simulink model "afe_dq_inv_psm"  (R2025a)
settings: Solver=ode1be  StartTime=0.0  StopTime=simlength  FixedStep=tc  MaxStep=tc
values from neighbouring files (symbols this model uses):
  Adrso = eye(2) + Arso*ts_afe    [init_model.m]
  b = tau_bez/omega_m_bez    [init_model.m]
  Crso = [1 0]    [init_model.m]
  CTRPIFF_CLIP_RELEASE = 0.001    [init_model.m]
  dead_time_AFE = 3e-6    (= 3e-06)    [init_model.m]
  dead_time_INV = 3e-6    (= 3e-06)    [init_model.m]
  deepNEGeta = 0.5    [init_model.m]
  deepNEGxi = 0    [init_model.m]
  deepPOSxi = 0.5    [init_model.m]
  emf_fb_p = 0.2    [init_model.m]
  emf_fb_p_ccaller_1 = emf_fb_p    (= 0.2)    [init_model.m]
  emf_fb_p_ccaller_2 = emf_fb_p    (= 0.2)    [init_model.m]
  emf_p = emf_fb_p*4/10    (= 0.08)    [init_model.m]
  emf_p_ccaller_1 = emf_fb_p_ccaller_1*4/10    (= 0.08)    [init_model.m]
  emf_p_ccaller_2 = emf_fb_p_ccaller_2*4/10    (= 0.08)    [init_model.m]
  fPWM_AFE = 4e3    (= 4000)    [init_model.m]
  fPWM_INV = fPWM_AFE    (= 4000)    [init_model.m]
  g0_500Hz = fcut_500Hz_flt * ts_afe * 2*pi    (= 0.392699081699)    [init_model.m]
  g1_500Hz = 1 - g0_500Hz    (= 0.607300918301)    [init_model.m]
  id_lim = 0.35    [init_model.m]
  Igrid_phase_normalization_factor = 270*sqrt(2)    [grid_emulator.m]    (also in init_model.m = 250e3/Vphase2/3/0.9*sqrt(2))
  iq_lim = 1.4    [init_model.m]
  ixi_pos_ref_lim = 1.6    [init_model.m]
  kg = Kobs(1)    [init_model.m]
  ki_afe = 45    [init_model.m]
  ki_i = 18    [init_model.m]
  ki_rc_grid = 35    [init_model.m]
  ki_vs = 35    [init_model.m]
  ki_w = 18    [init_model.m]
  kp_afe = 0.6    [init_model.m]
  kp_i = 0.25    [init_model.m]
  kp_rc_grid = 0.35    [init_model.m]
  kp_vs = 0.85    [init_model.m]
  kp_w = 2.5    [init_model.m]
  kw = Kobs(2)    [init_model.m]
  Ldrso = acker(Adrso',Crso',polesdrso)'    [init_model.m]
  motorc_m_scale = 2/3*Vdc_bez/ubez    [init_model.m]
  n1 = rms_perios/f_grid/ts_afe    [init_model.m]
  n10 = rms_perios/f_grid/ts_afe    [init_model.m]
  omega_grid_emulator_nom = w_grid    (= 314.159265359)    [grid_emulator.m]
  omega_grid_nom = w_grid    (= 314.159265359)    [grid_emulator.m]
  omega_m_sim = omega_m_bez    [init_model.m]
  pll_i1 = 80    [init_model.m]
  pll_i1_ddsrt = pll_i1/2    (= 40)    [init_model.m]
  pll_p = 1    [init_model.m]
  pll_p_ddsrt = pll_p/2    (= 0.5)    [init_model.m]
  pll_p_frt = 0.2    [init_model.m]
  simlength = 2    [init_model.m]
  start_time_LVRT = 2.0    (= 2)    [init_model.m]
  tc = ts_afe/200    (= 6.25e-07)    [init_model.m]
  time_aux_power_supply_fault = 1e3    (= 1000)    [init_model.m]
  time_phase_fault = 1e3    (= 1000)    [init_model.m]
  time_start_motor_control = 0.035    [init_model.m]
  ts_afe = 1/fPWM_AFE/2    (= 0.000125)    [init_model.m]
  ts_inv = 1/fPWM_INV/2    (= 0.000125)    [init_model.m]
  ugrid_factor = 1    [grid_emulator.m]
  V_phase_normalization_factor = Vgrid_phase_normalization_factor    [grid_emulator.m]
  Vdc_bez = 1070    [grid_emulator.m]
  Vdc_norm_ref = Vdc_ref/Vdc_nom    [init_model.m]
  Vdc_ref = 1070    [init_model.m]
  Vemu_ref_norm = Vemu_ref * sqrt(2) / V_phase_normalization_factor    [grid_emulator.m]
  Vgrid_phase_normalization_factor = Vphase2*sqrt(2)    [grid_emulator.m]    (also in init_model.m)
  vn_eta_pu = 0    [grid_emulator.m]
  vn_xi_pu = 0    [grid_emulator.m]
  vp_xi_pu = 1    [grid_emulator.m]
undefined symbols (not defined in the file or in its folder): Amplitude_U, Amplitude_V, Amplitude_W, end_time_LVRT, ibez, Jm, Ld_norm, Lq_norm, Ls_norm, magnitude, omega_bez, omega_m_bez, Phase_shift, psi_bez, psi_m, psi_m_norm, rpm_bez, rpm_torque_curve, Rs_norm, t_ramp, tau_bez, torque_torque_curve
libraries: fl_lib x114, nesl_utility x78, cstblocks x14, single_phase_transformer_lib x3, threephase_inductor_lib x2, simulink x2, flexshaft_lib x1, pmsm_uvw_with_harmonics_lib x1
(part 1 of 8)
settings Model: SimulationMode=accelerator  Creator=dbagn  LastModifiedBy=dbagn
settings SolverCC: NumberNewtonIterations=3.0  ZeroCrossControl=DisableAll  AlgebraicLoopSolver=TrustRegion  SolverResetMethod=Robust
settings DataIOCC: ReturnWorkspaceOutputs=off
settings OptimizationCC: ReuseModelBlockBuffer=off
settings DebuggingCC: UnconnectedInputMsg=warning  UnconnectedOutputMsg=warning  UnconnectedLineMsg=warning
settings ModelReferenceCC: EnableRefExpFcnMdlSchedulingChecks=on
settings SFSimCC: CustomCodeUndefinedFunction=ThrowError
settings SFSimCC: SimCustomHeaderCode=|
  | #include "mavgflt.h"
  | #include "mavgflt_simulink.h"
  | #include "bemf_obsv.h"
  | #include "bemf_obsv_simulink.h"
  | #include "bemf_obsv_load_est.h"
  | #include "bemf_obsv_load_est_simulink.h"
  | #include "dqvector_pi.h"
  | #include "dqvector_pi_simulink.h"
  | #include "sv_pwm_simulink.h"
  | #include "sv_pwm.h"
  | #include "first_harmonic_tracker.h"
  | #include "first_harmonic_tracker_simulink.h"
  | #include "dqpll_thyr.h"
  | #include "dqpll_thyr_simulink.h"
  | #include "dqpll_grid.h"
  | #include "dqpll_grid_simulink.h"
settings SFSimCC: SimUserSources=|
  | "mavgflt_simulink.c"
  | "mavgflt.c"
  | "bemf_obsv_simulink.c"
  | "bemf_obsv.c"
  | "bemf_obsv_load_est_simulink.c"
  | "bemf_obsv_load_est.c"
  | "dqvector_pi.c"
  | "dqvector_pi_simulink.c"
  | "sv_pwm_simulink.c"
  | "sv_pwm.c"
  | "first_harmonic_tracker_simulink.c"
  | "first_harmonic_tracker.c"
  | "dqpll_thyr_simulink.c"
  | "dqpll_thyr.c"
  | "dqpll_grid_simulink.c"
  | "dqpll_grid.c"
settings SFSimCC: SimUserIncludeDirs=|
  | include
  | src
settings RTWCC: GPUComputeCapability=3.5  DLArmComputeVersion=19.05

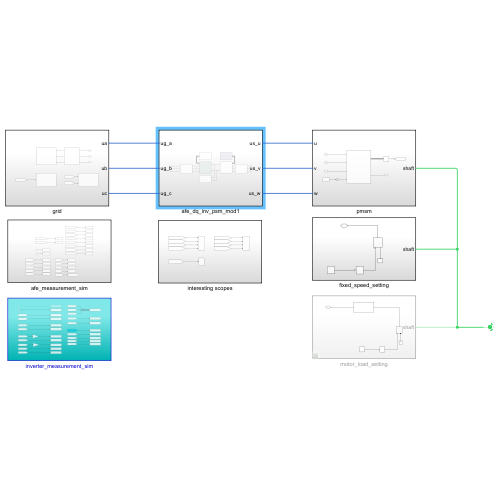
[thumbnail: Simulink's stored preview of the top-level diagram]
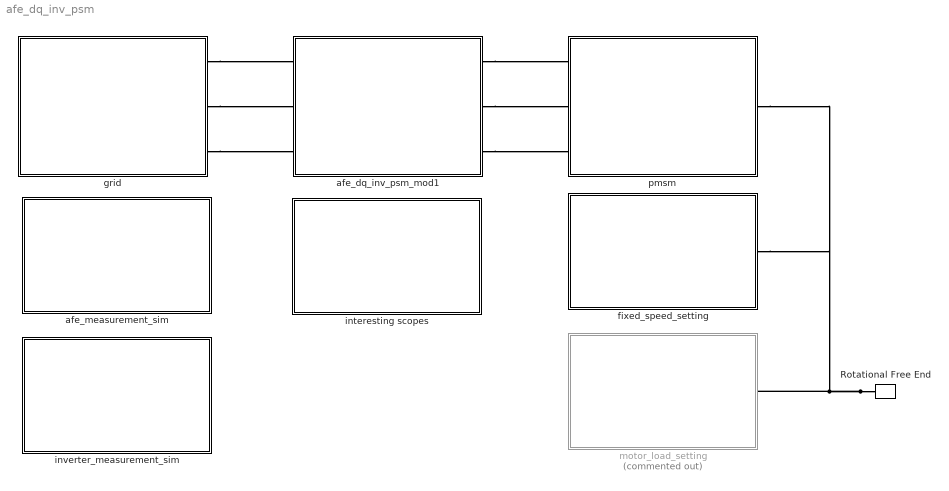
== system afe_dq_inv_psm ==
  Rotational Free End : fl_lib/Mechanical/Rotational Elements/Rotational Free End  w_specify=off  w_priority=None  w=0 rad/s  w_nominal_specify=off  w_nominal_value=1  w_nominal_unit=rad/s
  afe_dq_inv_psm_mod1 : Subsystem
  afe_measurement_sim : Subsystem
  fixed_speed_setting : Subsystem
  grid : Subsystem
  interesting scopes : Subsystem
  inverter_measurement_sim : Subsystem
  motor_load_setting : Subsystem  Commented=on
  pmsm : Subsystem
  connections:
  Rotational Free End/LConn1 -- pmsm/RConn1 -- fixed_speed_setting/LConn1 -- motor_load_setting/LConn1
  grid/RConn1 -- afe_dq_inv_psm_mod1/LConn1
  afe_dq_inv_psm_mod1/RConn1 -- pmsm/LConn1
  grid/RConn2 -- afe_dq_inv_psm_mod1/LConn2
  afe_dq_inv_psm_mod1/RConn2 -- pmsm/LConn2
  grid/RConn3 -- afe_dq_inv_psm_mod1/LConn3
  afe_dq_inv_psm_mod1/RConn3 -- pmsm/LConn3

== system afe_dq_inv_psm/afe_dq_inv_psm_mod1 ==
  LCL_filter : Subsystem
  L_filter : Subsystem
  afe : Subsystem
  afe_control : Subsystem
  brake : Subsystem
  inverter : Subsystem
  inverter_control : Subsystem
  ug_a : PMIOPort  Side=Left
  us_u : PMIOPort  Port=2  Side=Right
  ug_b : PMIOPort  Port=3  Side=Left
  us_v : PMIOPort  Port=4  Side=Right
  ug_c : PMIOPort  Port=5  Side=Left
  us_w : PMIOPort  Port=6  Side=Right
  wires:
  inverter_control/1(uab) -> inverter/1(uab)
  afe_control/1(uab_out) -> afe/1(uab)
  connections:
  L_filter/LConn2 -- inverter/LConn2
  inverter/RConn2 -- brake/LConn2 -- afe/RConn2
  inverter/RConn1 -- brake/LConn1 -- afe/RConn1
  L_filter/LConn1 -- inverter/LConn1
  L_filter/LConn3 -- inverter/LConn3
  L_filter/RConn2 -- us_v/RConn1
  L_filter/RConn3 -- us_w/RConn1
  L_filter/RConn1 -- us_u/RConn1
  LCL_filter/LConn1 -- afe/LConn1
  LCL_filter/LConn2 -- afe/LConn2
  LCL_filter/LConn3 -- afe/LConn3
  ug_a/RConn1 -- LCL_filter/RConn1
  ug_b/RConn1 -- LCL_filter/RConn2
  ug_c/RConn1 -- LCL_filter/RConn3

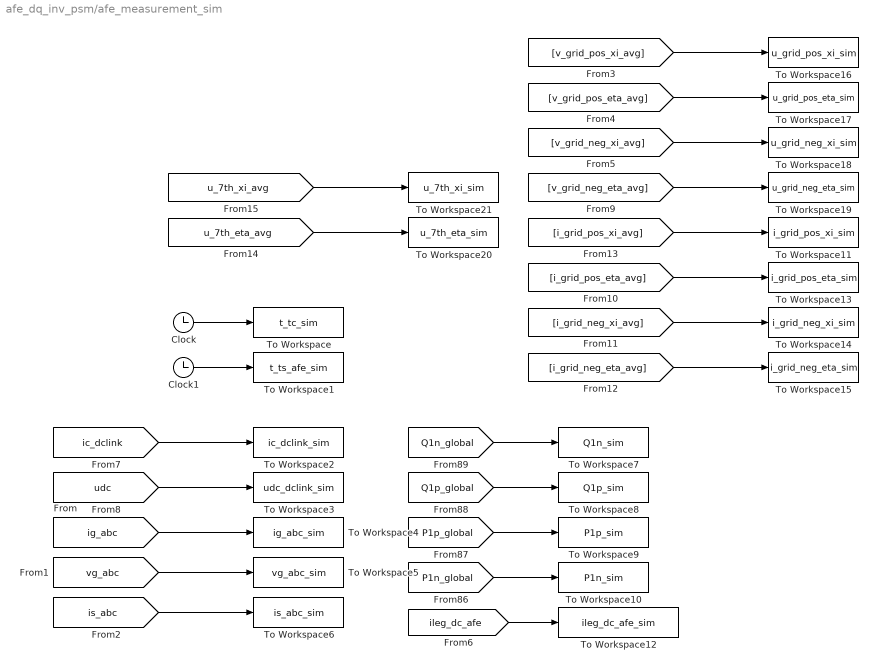
== system afe_dq_inv_psm/afe_measurement_sim ==
  Clock : Clock
  Clock1 : Clock
  To Workspace : ToWorkspace  VariableName=t_tc_sim  SampleTime=tc
      settings: MaxDataPoints=Nc
  To Workspace1 : ToWorkspace  VariableName=t_ts_afe_sim  SampleTime=ts_afe
      settings: MaxDataPoints=Ns_afe
  To Workspace10 : ToWorkspace  VariableName=P1n_sim  SampleTime=ts_afe
      settings: MaxDataPoints=Ns_afe
  To Workspace11 : ToWorkspace  VariableName=i_grid_pos_xi_sim  SampleTime=ts_afe
      settings: MaxDataPoints=Ns_afe
  To Workspace12 : ToWorkspace  VariableName=ileg_dc_afe_sim  SampleTime=tc
      settings: MaxDataPoints=Nc
  To Workspace13 : ToWorkspace  VariableName=i_grid_pos_eta_sim  SampleTime=ts_afe
      settings: MaxDataPoints=Ns_afe
  To Workspace14 : ToWorkspace  VariableName=i_grid_neg_xi_sim  SampleTime=ts_afe
      settings: MaxDataPoints=Ns_afe
  To Workspace15 : ToWorkspace  VariableName=i_grid_neg_eta_sim  SampleTime=ts_afe
      settings: MaxDataPoints=Ns_afe
  To Workspace16 : ToWorkspace  VariableName=u_grid_pos_xi_sim  SampleTime=ts_afe
      settings: MaxDataPoints=Ns_afe
  To Workspace17 : ToWorkspace  VariableName=u_grid_pos_eta_sim  SampleTime=ts_afe
      settings: MaxDataPoints=Ns_afe
  To Workspace18 : ToWorkspace  VariableName=u_grid_neg_xi_sim  SampleTime=ts_afe
      settings: MaxDataPoints=Ns_afe
  To Workspace19 : ToWorkspace  VariableName=u_grid_neg_eta_sim  SampleTime=ts_afe
      settings: MaxDataPoints=Ns_afe
  To Workspace2 : ToWorkspace  VariableName=ic_dclink_sim  SampleTime=tc
      settings: MaxDataPoints=Nc
  To Workspace20 : ToWorkspace  VariableName=u_7th_eta_sim  SampleTime=ts_afe
      settings: MaxDataPoints=Ns_afe
  To Workspace21 : ToWorkspace  VariableName=u_7th_xi_sim  SampleTime=ts_afe
      settings: MaxDataPoints=Ns_afe
  To Workspace3 : ToWorkspace  VariableName=udc_dclink_sim  SampleTime=tc
      settings: MaxDataPoints=Nc
  To Workspace4 : ToWorkspace  VariableName=ig_abc_sim  SampleTime=tc
      settings: MaxDataPoints=Nc
  To Workspace5 : ToWorkspace  VariableName=vg_abc_sim  SampleTime=tc
      settings: MaxDataPoints=Nc
  To Workspace6 : ToWorkspace  VariableName=is_abc_sim  SampleTime=tc
      settings: MaxDataPoints=Nc
  To Workspace7 : ToWorkspace  VariableName=Q1n_sim  SampleTime=ts_afe
      settings: MaxDataPoints=Ns_afe
  To Workspace8 : ToWorkspace  VariableName=Q1p_sim  SampleTime=ts_afe
      settings: MaxDataPoints=Ns_afe
  To Workspace9 : ToWorkspace  VariableName=P1p_sim  SampleTime=ts_afe
      settings: MaxDataPoints=Ns_afe
  wires:
  Clock1/1 -> To Workspace1/1
  Clock/1 -> To Workspace/1
  [ic_dclink] -> To Workspace2/1
  [udc] -> To Workspace3/1
  [ig_abc] -> To Workspace4/1
  [vg_abc] -> To Workspace5/1
  [is_abc] -> To Workspace6/1
  [Q1n_global] -> To Workspace7/1
  [Q1p_global] -> To Workspace8/1
  [P1p_global] -> To Workspace9/1
  [P1n_global] -> To Workspace10/1
  [ileg_dc_afe] -> To Workspace12/1
  [i_grid_pos_xi_avg] -> To Workspace11/1
  [i_grid_pos_eta_avg] -> To Workspace13/1
  [i_grid_neg_xi_avg] -> To Workspace14/1
  [i_grid_neg_eta_avg] -> To Workspace15/1
  [v_grid_pos_xi_avg] -> To Workspace16/1
  [v_grid_pos_eta_avg] -> To Workspace17/1
  [v_grid_neg_xi_avg] -> To Workspace18/1
  [v_grid_neg_eta_avg] -> To Workspace19/1
  [u_7th_eta_avg] -> To Workspace20/1
  [u_7th_xi_avg] -> To Workspace21/1

== system afe_dq_inv_psm/fixed_speed_setting ==
  Ideal Angular Velocity Source : fl_lib/Mechanical/Mechanical Sources/Ideal Angular Velocity Source
  Mechanical Rotational Reference : fl_lib/Mechanical/Rotational Elements/Mechanical Rotational Reference
  PS Step1 : fl_lib/Physical Signals/Sources/PS Step  step_time=0.025 s  initial_value=0 rpm  final_value=rpm_sim rpm
  PS Transfer Function : fl_lib/Physical Signals/Linear Operators/PS Transfer Function  transfer_function_type=foundation.enum.transfer_function_type.lag  T=0.1 s  T1=2 s  T2=1 s  reset_method=foundation.enum.IntegratorResetSpec.None  initial_condition_spec=foundation.enum.IntegratorICSpec.Internal  y0=0 rpm
      settings: InternalSimscapePortConfiguration="{\"Bottom\":[],\"Left\":[{\"id\":\"U\",\"label\":\"\",\"type\":\"input\"}],\"Right\":[{\"id\":\"Y\",\"label\":\"\",\"type\":\"output\"}],\"Top\":[]}"
  shaft : PMIOPort  Side=Left
  connections:
  Mechanical Rotational Reference/LConn1 -- Ideal Angular Velocity Source/RConn2
  Ideal Angular Velocity Source/LConn1 -- shaft/RConn1
  PS Step1/RConn1 -- PS Transfer Function/LConn1
  PS Transfer Function/RConn1 -- Ideal Angular Velocity Source/RConn1

== system afe_dq_inv_psm/grid ==
  grid_emulator : Subsystem
  instantaneus_power : Subsystem
  sequences : Subsystem
  threephase_vi_measures : Subsystem
  ua : PMIOPort  Side=Right
  ub : PMIOPort  Port=2  Side=Right
  uc : PMIOPort  Port=3  Side=Right
  wires:
  [gamma_grid_pll] -> sequences/1(wt)
  [vg_abc] -> instantaneus_power/1(Vline)
  [ig_abc] -> instantaneus_power/2(Iline)
  connections:
  threephase_vi_measures/LConn3 -- grid_emulator/RConn3
  threephase_vi_measures/LConn1 -- grid_emulator/RConn1
  threephase_vi_measures/RConn2 -- ub/RConn1
  threephase_vi_measures/LConn2 -- grid_emulator/RConn2
  threephase_vi_measures/RConn1 -- ua/RConn1
  threephase_vi_measures/RConn3 -- uc/RConn1

== system afe_dq_inv_psm/interesting scopes ==
  current_sequences : Scope  NumInputPorts=4
      settings: SampleTime=ts_afe  ActiveDisplayYMinimum=-1.81849  ActiveDisplayYMaximum=0.36458  DataLoggingVariableName=ScopeData2
  i_grid_seq_ref : Scope
      settings: SampleTime=ts_afe  ActiveDisplayYMinimum=-1.125  ActiveDisplayYMaximum=0.125
  voltage_sequences : Scope  NumInputPorts=4
      settings: SampleTime=ts_afe  ActiveDisplayYMinimum=-0.75427  ActiveDisplayYMaximum=1.21467
  wires:
  [v_grid_neg_eta_avg] -> voltage_sequences/4  "u_grid_neg_eta"
  [i_grid_neg_xi_avg] -> current_sequences/3  "i_grid_neg_xi"
  [v_grid_pos_eta_avg] -> voltage_sequences/2  "u_grid_pos_eta"
  [v_grid_neg_xi_avg] -> voltage_sequences/3  "u_grid_neg_xi"
  [i_grid_pos_xi_avg] -> current_sequences/1  "i_grid_pos_xi"
  [i_grid_neg_eta_avg] -> current_sequences/4  "i_grid_neg_eta"
  [v_grid_pos_xi_avg] -> voltage_sequences/1  "u_grid_pos_xi"
  [i_grid_pos_eta_avg] -> current_sequences/2  "i_grid_pos_eta"
  [i_grid_seq_ref] -> i_grid_seq_ref/1  "i_grid_seq_ref"

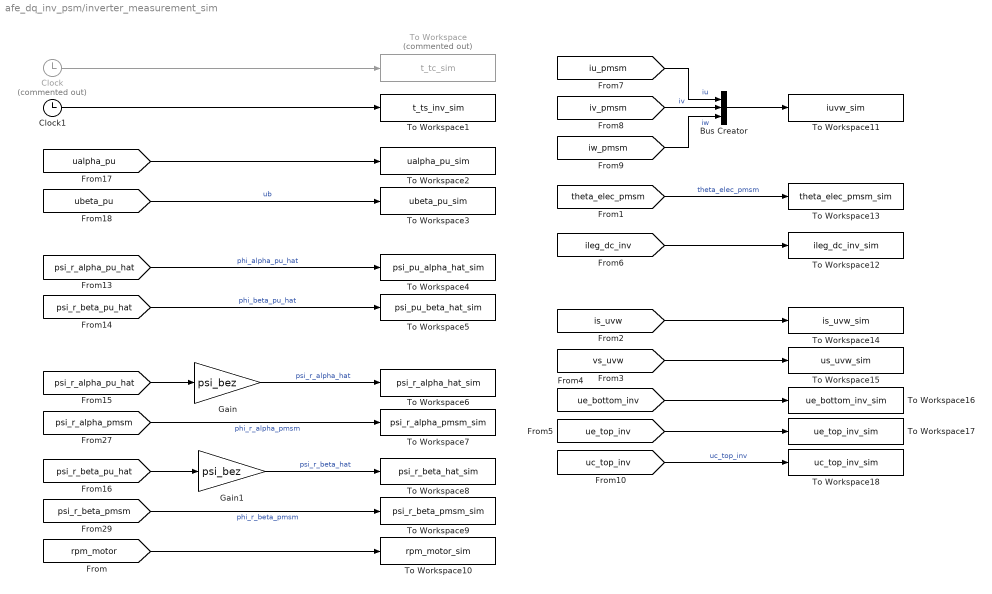
== system afe_dq_inv_psm/inverter_measurement_sim ==
  Bus Creator : BusCreator  Inputs=3
  Clock : Clock  Commented=on
  Clock1 : Clock
  Gain : Gain  Gain=psi_bez
  Gain1 : Gain  Gain=psi_bez
  To Workspace : ToWorkspace  Commented=on  VariableName=t_tc_sim  SampleTime=tc
      settings: MaxDataPoints=Nc
  To Workspace1 : ToWorkspace  VariableName=t_ts_inv_sim  SampleTime=ts_inv
      settings: MaxDataPoints=Ns_inv
  To Workspace10 : ToWorkspace  VariableName=rpm_motor_sim  SampleTime=ts_inv
      settings: MaxDataPoints=Ns_inv
  To Workspace11 : ToWorkspace  VariableName=iuvw_sim  SampleTime=tc
      settings: MaxDataPoints=Nc
  To Workspace12 : ToWorkspace  VariableName=ileg_dc_inv_sim  SampleTime=tc
      settings: MaxDataPoints=Nc
  To Workspace13 : ToWorkspace  VariableName=theta_elec_pmsm_sim  SampleTime=ts_inv
      settings: MaxDataPoints=Ns_inv
  To Workspace14 : ToWorkspace  VariableName=is_uvw_sim  SampleTime=tc
      settings: MaxDataPoints=Nc
  To Workspace15 : ToWorkspace  VariableName=us_uvw_sim  SampleTime=tc
      settings: MaxDataPoints=Nc
  To Workspace16 : ToWorkspace  VariableName=ue_bottom_inv_sim  SampleTime=tc
      settings: MaxDataPoints=Nc
  To Workspace17 : ToWorkspace  VariableName=ue_top_inv_sim  SampleTime=tc
      settings: MaxDataPoints=Nc
  To Workspace18 : ToWorkspace  VariableName=uc_top_inv_sim  SampleTime=tc
      settings: MaxDataPoints=Nc
  To Workspace2 : ToWorkspace  VariableName=ualpha_pu_sim  SampleTime=ts_inv
      settings: MaxDataPoints=Ns_inv
  To Workspace3 : ToWorkspace  VariableName=ubeta_pu_sim  SampleTime=ts_inv
      settings: MaxDataPoints=Ns_inv
  To Workspace4 : ToWorkspace  VariableName=psi_pu_alpha_hat_sim  SampleTime=ts_inv
      settings: MaxDataPoints=Ns_inv
  To Workspace5 : ToWorkspace  VariableName=psi_pu_beta_hat_sim  SampleTime=ts_inv
      settings: MaxDataPoints=Ns_inv
  To Workspace6 : ToWorkspace  VariableName=psi_r_alpha_hat_sim  SampleTime=ts_inv
      settings: MaxDataPoints=Ns_inv
  To Workspace7 : ToWorkspace  VariableName=psi_r_alpha_pmsm_sim  SampleTime=ts_inv
      settings: MaxDataPoints=Ns_inv
  To Workspace8 : ToWorkspace  VariableName=psi_r_beta_hat_sim  SampleTime=ts_inv
      settings: MaxDataPoints=Ns_inv
  To Workspace9 : ToWorkspace  VariableName=psi_r_beta_pmsm_sim  SampleTime=ts_inv
      settings: MaxDataPoints=Ns_inv
  wires:
  [psi_r_beta_pu_hat] -> Gain1/1
  Gain1/1 -> To Workspace8/1  "psi_r_beta_hat"
  [psi_r_beta_pu_hat] -> To Workspace5/1  "phi_beta_pu_hat"
  [psi_r_alpha_pu_hat] -> To Workspace4/1  "phi_alpha_pu_hat"
  [ualpha_pu] -> To Workspace2/1
  [psi_r_alpha_pmsm] -> To Workspace7/1  "phi_r_alpha_pmsm"
  Clock1/1 -> To Workspace1/1
  Gain/1 -> To Workspace6/1  "psi_r_alpha_hat"
  Clock/1 -> To Workspace/1
  [ubeta_pu] -> To Workspace3/1  "ub"
  [psi_r_alpha_pu_hat] -> Gain/1
  [psi_r_beta_pmsm] -> To Workspace9/1  "phi_r_beta_pmsm"
  [rpm_motor] -> To Workspace10/1
  [iv_pmsm] -> Bus Creator/2  "iv"
  [iw_pmsm] -> Bus Creator/3  "iw"
  [iu_pmsm] -> Bus Creator/1  "iu"
  Bus Creator/1 -> To Workspace11/1
  [theta_elec_pmsm] -> To Workspace13/1  "theta_elec_pmsm"
  [ileg_dc_inv] -> To Workspace12/1
  [is_uvw] -> To Workspace14/1
  [vs_uvw] -> To Workspace15/1
  [ue_bottom_inv] -> To Workspace16/1
  [ue_top_inv] -> To Workspace17/1
  [uc_top_inv] -> To Workspace18/1  "uc_top_inv"

== system afe_dq_inv_psm/motor_load_setting ==
  Ideal Torque Source : fl_lib/Mechanical/Mechanical Sources/Ideal Torque Source
  Mechanical Rotational Reference : fl_lib/Mechanical/Rotational Elements/Mechanical Rotational Reference
  PS Step : fl_lib/Physical Signals/Sources/PS Step  step_time=0.25 s  initial_value=1 N*m  final_value=tau_bez N*m
  PS Transfer Function : fl_lib/Physical Signals/Linear Operators/PS Transfer Function  transfer_function_type=foundation.enum.transfer_function_type.lag  T=1 s  T1=2 s  T2=1 s  reset_method=foundation.enum.IntegratorResetSpec.None  initial_condition_spec=foundation.enum.IntegratorICSpec.Internal  y0=0 N*m
      settings: InternalSimscapePortConfiguration="{\"Bottom\":[],\"Left\":[{\"id\":\"U\",\"label\":\"\",\"type\":\"input\"}],\"Right\":[{\"id\":\"Y\",\"label\":\"\",\"type\":\"output\"}],\"Top\":[]}"
  flex-shaft : Subsystem
      mask Display: disp('flexible shaft')
  shaft : PMIOPort  Side=Left
  connections:
  Ideal Torque Source/LConn1 -- flex-shaft/RConn1
  Ideal Torque Source/RConn2 -- Mechanical Rotational Reference/LConn1
  PS Transfer Function/RConn1 -- Ideal Torque Source/RConn1
  PS Step/RConn1 -- PS Transfer Function/LConn1
  flex-shaft/LConn1 -- shaft/RConn1

== system afe_dq_inv_psm/pmsm ==
  Constant : Constant  Value=psi_m
  Selector : Selector  InputPortWidth=19  IndexOptions=Index vector (dialog)  Indices=16  OutputSizes=1
  Simulink-PS Converter3 : nesl_utility/Simulink-PS Converter  PhysicalDomain=network_engine_domain  SubClassName=ps_input  LeftPortType=input  RightPortType=output  PseudoPeriodic=off  Frequencies=[]  NoiseDistribution=none  NoiseParameters=[]  Unit=V*s  AffineConversion=on  FilteringAndDerivatives=provide  SimscapeFilterOrder=1  InputFilterTimeConstant=0.001  UdotUserProvided=0
  synchronous_motor : Subsystem
  u : PMIOPort  Side=Left
  v : PMIOPort  Port=2  Side=Left
  w : PMIOPort  Port=3  Side=Left
  shaft : PMIOPort  Port=4  Side=Right
  tag scope: rpm_motor=global
  wires:
  synchronous_motor/1(motor_data) -> Selector/1
  Selector/1 -> [rpm_motor]
  Constant/1 -> Simulink-PS Converter3/1
  connections:
  synchronous_motor/LConn1 -- u/RConn1
  Simulink-PS Converter3/RConn1 -- synchronous_motor/LConn4
  synchronous_motor/LConn3 -- w/RConn1
  synchronous_motor/LConn2 -- v/RConn1
  shaft/RConn1 -- synchronous_motor/RConn1

== system afe_dq_inv_psm/afe_dq_inv_psm_mod1/LCL_filter ==
  CFu1 : fl_lib/Electrical/Electrical Elements/Capacitor  c=CFu F  r=RCFu Ohm  g=0 1/Ohm  i_specify=off  i_priority=None  i=0 A  i_nominal_specify=off  i_nominal_value=1  i_nominal_unit=A  v_specify=off  v_priority=None  v=0 V  v_nominal_specify=off  v_nominal_value=1  v_nominal_unit=V  vc_specify=off  vc_priority=High  vc=0 V  vc_nominal_specify=off  vc_nominal_value=1  vc_nominal_unit=V
  CFu2 : fl_lib/Electrical/Electrical Elements/Capacitor  c=CFu F  r=RCFu Ohm  g=0 1/Ohm  i_specify=off  i_priority=None  i=0 A  i_nominal_specify=off  i_nominal_value=1  i_nominal_unit=A  v_specify=off  v_priority=None  v=0 V  v_nominal_specify=off  v_nominal_value=1  v_nominal_unit=V  vc_specify=off  vc_priority=High  vc=0 V  vc_nominal_specify=off  vc_nominal_value=1  vc_nominal_unit=V
  CFu3 : fl_lib/Electrical/Electrical Elements/Capacitor  c=CFu F  r=RCFu Ohm  g=0 1/Ohm  i_specify=off  i_priority=None  i=0 A  i_nominal_specify=off  i_nominal_value=1  i_nominal_unit=A  v_specify=off  v_priority=None  v=0 V  v_nominal_specify=off  v_nominal_value=1  v_nominal_unit=V  vc_specify=off  vc_priority=High  vc=0 V  vc_nominal_specify=off  vc_nominal_value=1  vc_nominal_unit=V
  Inductor : fl_lib/Electrical/Electrical Elements/Inductor  l=1e-6 H  r=0 Ohm  g=1e-9 1/Ohm  i_specify=on  i_priority=High  i=0 A  i_nominal_specify=off  i_nominal_value=1  i_nominal_unit=A  v_specify=off  v_priority=None  v=0 V  v_nominal_specify=off  v_nominal_value=1  v_nominal_unit=V  i_L_specify=off  i_L_priority=High  i_L=0 A  i_L_nominal_specify=off  i_L_nominal_value=1  i_L_nominal_unit=A
  Inductor1 : fl_lib/Electrical/Electrical Elements/Inductor  l=1e-6 H  r=0 Ohm  g=1e-9 1/Ohm  i_specify=on  i_priority=High  i=0 A  i_nominal_specify=off  i_nominal_value=1  i_nominal_unit=A  v_specify=off  v_priority=None  v=0 V  v_nominal_specify=off  v_nominal_value=1  v_nominal_unit=V  i_L_specify=off  i_L_priority=High  i_L=0 A  i_L_nominal_specify=off  i_L_nominal_value=1  i_L_nominal_unit=A
  Inductor2 : fl_lib/Electrical/Electrical Elements/Inductor  l=1e-6 H  r=0 Ohm  g=1e-9 1/Ohm  i_specify=on  i_priority=High  i=0 A  i_nominal_specify=off  i_nominal_value=1  i_nominal_unit=A  v_specify=off  v_priority=None  v=0 V  v_nominal_specify=off  v_nominal_value=1  v_nominal_unit=V  i_L_specify=off  i_L_priority=High  i_L=0 A  i_L_nominal_specify=off  i_L_nominal_value=1  i_L_nominal_unit=A
  threephase inductor : threephase_inductor_lib/threephase inductor  Lp=LFu1_AFE H  L0=LFu1_AFE_0 H  Rp=2.4e-3 Ohm  R0=0.8e-3 Ohm  Lls=5e-6 H  uu_1_specify=off  uu_1_priority=None  uu_1=0 V  uu_1_nominal_specify=off  uu_1_nominal_unit=V  uu_1_nominal_value=1  uv_1_specify=off  uv_1_priority=None  uv_1=0 V  uv_1_nominal_specify=off  uv_1_nominal_unit=V  uv_1_nominal_value=1  uw_1_specify=off  uw_1_priority=None  uw_1=0 V  uw_1_nominal_specify=off  uw_1_nominal_unit=V  uw_1_nominal_value=1  uu_2_specify=off  uu_2_priority=None  uu_2=0 V  uu_2_nominal_specify=off  uu_2_nominal_unit=V  uu_2_nominal_value=1  uv_2_specify=off  uv_2_priority=None  uv_2=0 V  uv_2_nominal_specify=off  uv_2_nominal_unit=V  uv_2_nominal_value=1  uw_2_specify=off  uw_2_priority=None  uw_2=0 V  uw_2_nominal_specify=off  uw_2_nominal_unit=V  uw_2_nominal_value=1  iu_specify=off  iu_priority=High  iu=0 A  iu_nominal_specify=off  iu_nominal_unit=A  iu_nominal_value=1  iv_specify=off  iv_priority=High  iv=0 A  iv_nominal_specify=off  iv_nominal_unit=A  iv_nominal_value=1  iw_specify=off  iw_priority=High  iw=0 A  iw_nominal_specify=off  iw_nominal_unit=A  iw_nominal_value=1
      settings: InternalSimscapePortConfiguration="{\"Bottom\":[],\"Left\":[{\"id\":\"up1\",\"label\":\"u1\",\"type\":\"foundation.electrical.electrical\"},{\"id\":\"vp1\",\"label\":\"v1\",\"type\":\"foundation.electrical.electrical\"},{\"id\":\"wp1\",\"label\":\"w1\",\"type\":\"foundation.electrical.electrical\"}],\"Right\":[{\"id\":\"up2\",\"label\":\"u2\",\"type\":\"foundation.electrical.electrical\"},{\"id\":\"vp2\",\"label\":\"v2\",\"type\":\"foundation.electrical.electrical\"},{\"id\":\"wp2\",\"label\":\"w2\",\"type\":\"foundation.electrical.electrical\"}],\"Top\":[]}"
  threephase_vi_measures_stack : Subsystem
  us_a : PMIOPort  Side=Left
  ug_a : PMIOPort  Port=2  Side=Right
  us_b : PMIOPort  Port=3  Side=Left
  ug_b : PMIOPort  Port=4  Side=Right
  us_c : PMIOPort  Port=5  Side=Left
  ug_c : PMIOPort  Port=6  Side=Right
  connections:
  CFu3/RConn1 -- CFu2/RConn1 -- CFu1/RConn1
  CFu1/LConn1 -- Inductor/RConn1 -- ug_a/RConn1
  ug_c/RConn1 -- Inductor2/RConn1 -- CFu3/LConn1
  CFu2/LConn1 -- Inductor1/RConn1 -- ug_b/RConn1
  threephase_vi_measures_stack/LConn1 -- us_a/RConn1
  threephase_vi_measures_stack/LConn2 -- us_b/RConn1
  threephase_vi_measures_stack/LConn3 -- us_c/RConn1
  threephase_vi_measures_stack/RConn1 -- threephase inductor/LConn1
  threephase_vi_measures_stack/RConn2 -- threephase inductor/LConn2
  threephase_vi_measures_stack/RConn3 -- threephase inductor/LConn3
  threephase inductor/RConn1 -- Inductor/LConn1
  Inductor1/LConn1 -- threephase inductor/RConn2
  Inductor2/LConn1 -- threephase inductor/RConn3

== system afe_dq_inv_psm/afe_dq_inv_psm_mod1/L_filter ==
  Inductor : fl_lib/Electrical/Electrical Elements/Inductor  l=1e-6 H  r=0 Ohm  g=1e-9 1/Ohm  i_specify=off  i_priority=None  i=0 A  i_nominal_specify=off  i_nominal_value=1  i_nominal_unit=A  v_specify=off  v_priority=None  v=0 V  v_nominal_specify=off  v_nominal_value=1  v_nominal_unit=V  i_L_specify=off  i_L_priority=High  i_L=0 A  i_L_nominal_specify=off  i_L_nominal_value=1  i_L_nominal_unit=A
  Inductor1 : fl_lib/Electrical/Electrical Elements/Inductor  l=1e-6 H  r=0 Ohm  g=1e-9 1/Ohm  i_specify=off  i_priority=None  i=0 A  i_nominal_specify=off  i_nominal_value=1  i_nominal_unit=A  v_specify=off  v_priority=None  v=0 V  v_nominal_specify=off  v_nominal_value=1  v_nominal_unit=V  i_L_specify=off  i_L_priority=High  i_L=0 A  i_L_nominal_specify=off  i_L_nominal_value=1  i_L_nominal_unit=A
  Inductor2 : fl_lib/Electrical/Electrical Elements/Inductor  l=1e-6 H  r=0 Ohm  g=1e-9 1/Ohm  i_specify=off  i_priority=None  i=0 A  i_nominal_specify=off  i_nominal_value=1  i_nominal_unit=A  v_specify=off  v_priority=None  v=0 V  v_nominal_specify=off  v_nominal_value=1  v_nominal_unit=V  i_L_specify=off  i_L_priority=High  i_L=0 A  i_L_nominal_specify=off  i_L_nominal_value=1  i_L_nominal_unit=A
  threephase inductor : threephase_inductor_lib/threephase inductor  Lp=LFi H  L0=5e-6 H  Rp=2.4e-3 Ohm  R0=0.8e-3 Ohm  Lls=5e-6 H  uu_1_specify=off  uu_1_priority=None  uu_1=0 V  uu_1_nominal_specify=off  uu_1_nominal_unit=V  uu_1_nominal_value=1  uv_1_specify=off  uv_1_priority=None  uv_1=0 V  uv_1_nominal_specify=off  uv_1_nominal_unit=V  uv_1_nominal_value=1  uw_1_specify=off  uw_1_priority=None  uw_1=0 V  uw_1_nominal_specify=off  uw_1_nominal_unit=V  uw_1_nominal_value=1  uu_2_specify=off  uu_2_priority=None  uu_2=0 V  uu_2_nominal_specify=off  uu_2_nominal_unit=V  uu_2_nominal_value=1  uv_2_specify=off  uv_2_priority=None  uv_2=0 V  uv_2_nominal_specify=off  uv_2_nominal_unit=V  uv_2_nominal_value=1  uw_2_specify=off  uw_2_priority=None  uw_2=0 V  uw_2_nominal_specify=off  uw_2_nominal_unit=V  uw_2_nominal_value=1  iu_specify=off  iu_priority=None  iu=0 A  iu_nominal_specify=off  iu_nominal_unit=A  iu_nominal_value=1  iv_specify=off  iv_priority=None  iv=0 A  iv_nominal_specify=off  iv_nominal_unit=A  iv_nominal_value=1  iw_specify=off  iw_priority=None  iw=0 A  iw_nominal_specify=off  iw_nominal_unit=A  iw_nominal_value=1
      settings: InternalSimscapePortConfiguration="{\"Bottom\":[],\"Left\":[{\"id\":\"up1\",\"label\":\"u1\",\"type\":\"foundation.electrical.electrical\"},{\"id\":\"vp1\",\"label\":\"v1\",\"type\":\"foundation.electrical.electrical\"},{\"id\":\"wp1\",\"label\":\"w1\",\"type\":\"foundation.electrical.electrical\"}],\"Right\":[{\"id\":\"up2\",\"label\":\"u2\",\"type\":\"foundation.electrical.electrical\"},{\"id\":\"vp2\",\"label\":\"v2\",\"type\":\"foundation.electrical.electrical\"},{\"id\":\"wp2\",\"label\":\"w2\",\"type\":\"foundation.electrical.electrical\"}],\"Top\":[]}"
  threephase_vi_measures_stack : Subsystem
  us_u : PMIOPort  Side=Left
  uu : PMIOPort  Port=2  Side=Right
  us_v : PMIOPort  Port=3  Side=Left
  uv : PMIOPort  Port=4  Side=Right
  us_w : PMIOPort  Port=5  Side=Left
  uw : PMIOPort  Port=6  Side=Right
  connections:
  threephase_vi_measures_stack/LConn1 -- us_u/RConn1
  threephase_vi_measures_stack/LConn2 -- us_v/RConn1
  threephase_vi_measures_stack/LConn3 -- us_w/RConn1
  threephase inductor/LConn1 -- threephase_vi_measures_stack/RConn1
  threephase inductor/LConn2 -- threephase_vi_measures_stack/RConn2
  threephase inductor/LConn3 -- threephase_vi_measures_stack/RConn3
  threephase inductor/RConn1 -- Inductor/LConn1
  threephase inductor/RConn2 -- Inductor1/LConn1
  threephase inductor/RConn3 -- Inductor2/LConn1
  Inductor/RConn1 -- uu/RConn1
  Inductor1/RConn1 -- uv/RConn1
  Inductor2/RConn1 -- uw/RConn1

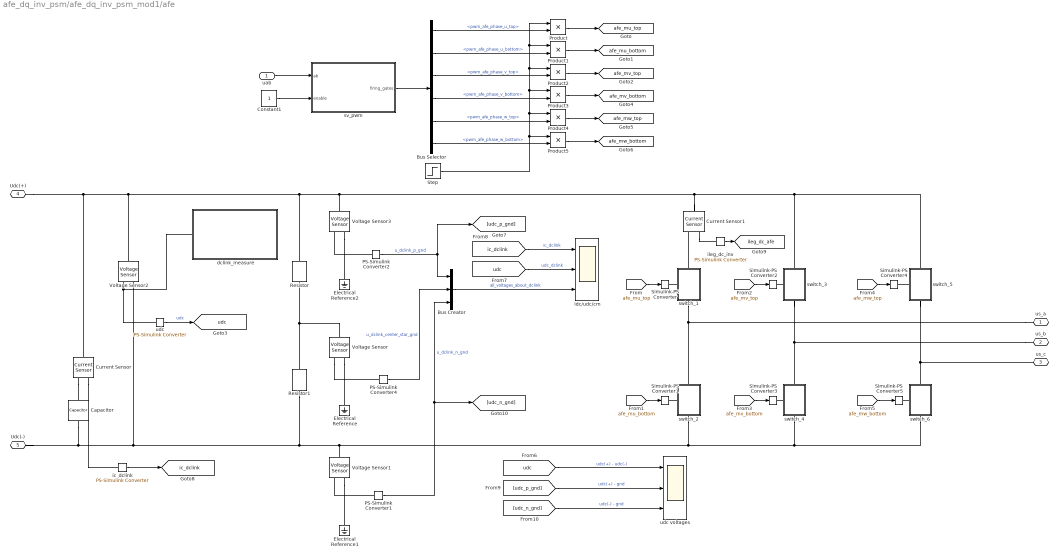
== system afe_dq_inv_psm/afe_dq_inv_psm_mod1/afe ==
  uab : Inport
  Bus Creator : BusCreator  Inputs=3
  Bus Selector : BusSelector  OutputSignals=pwm_afe_phase_u_top,pwm_afe_phase_u_bottom,pwm_afe_phase_v_top,pwm_afe_phase_v_bottom,pwm_afe_phase_w_top,pwm_afe_phase_w_bottom
  Capacitor : fl_lib/Electrical/Electrical Elements/Capacitor  c=CFi F  r=0.2e-3 Ohm  g=0 1/Ohm  i_specify=off  i_priority=None  i=0 A  i_nominal_specify=off  i_nominal_value=1  i_nominal_unit=A  v_specify=on  v_priority=High  v=Vdc_bez V  v_nominal_specify=off  v_nominal_value=1  v_nominal_unit=V  vc_specify=on  vc_priority=High  vc=Vdc_bez V  vc_nominal_specify=off  vc_nominal_value=1  vc_nominal_unit=V
  Constant1 : Constant
  Current Sensor : fl_lib/Electrical/Electrical Sensors/Current Sensor
  Current Sensor1 : fl_lib/Electrical/Electrical Sensors/Current Sensor
  Electrical Reference : fl_lib/Electrical/Electrical Elements/Electrical Reference
  Electrical Reference1 : fl_lib/Electrical/Electrical Elements/Electrical Reference
  Electrical Reference2 : fl_lib/Electrical/Electrical Elements/Electrical Reference
  PS-Simulink Converter1 : nesl_utility/PS-Simulink Converter  PhysicalDomain=network_engine_domain  SubClassName=ps_output  LeftPortType=input  RightPortType=output  PseudoPeriodic=off  Frequencies=[]  VectorFormat=1-D array  Unit=V  AffineConversion=on
  PS-Simulink Converter2 : nesl_utility/PS-Simulink Converter  PhysicalDomain=network_engine_domain  SubClassName=ps_output  LeftPortType=input  RightPortType=output  PseudoPeriodic=off  Frequencies=[]  VectorFormat=1-D array  Unit=V  AffineConversion=on
  PS-Simulink Converter4 : nesl_utility/PS-Simulink Converter  PhysicalDomain=network_engine_domain  SubClassName=ps_output  LeftPortType=input  RightPortType=output  PseudoPeriodic=off  Frequencies=[]  VectorFormat=1-D array  Unit=V  AffineConversion=on
  Product{,1..5} (6 alike) : Product
  Resistor : fl_lib/Electrical/Electrical Elements/Resistor  R=1e6 Ohm  i_specify=off  i_priority=None  i=0 A  i_nominal_specify=off  i_nominal_value=1  i_nominal_unit=A  v_specify=off  v_priority=None  v=0 V  v_nominal_specify=off  v_nominal_value=1  v_nominal_unit=V
  Resistor1 : fl_lib/Electrical/Electrical Elements/Resistor  R=1e6 Ohm  i_specify=off  i_priority=None  i=0 A  i_nominal_specify=off  i_nominal_value=1  i_nominal_unit=A  v_specify=off  v_priority=None  v=0 V  v_nominal_specify=off  v_nominal_value=1  v_nominal_unit=V
  Simulink-PS Converter{,1..5} (6 alike) : nesl_utility/Simulink-PS Converter  PhysicalDomain=network_engine_domain  SubClassName=ps_input  LeftPortType=input  RightPortType=output  PseudoPeriodic=off  Frequencies=[]  NoiseDistribution=none  NoiseParameters=[]  Unit=1  AffineConversion=off  FilteringAndDerivatives=provide  SimscapeFilterOrder=1  InputFilterTimeConstant=0.001  UdotUserProvided=0
  Step : Step  Time=time_aux_power_supply_fault  Before=1  After=0  SampleTime=0
  Voltage Sensor{,1..3} (4 alike) : fl_lib/Electrical/Electrical Sensors/Voltage Sensor
  dclink_measure : Subsystem
  ic_dclink : nesl_utility/PS-Simulink Converter  PhysicalDomain=network_engine_domain  SubClassName=ps_output  LeftPortType=input  RightPortType=output  PseudoPeriodic=off  Frequencies=[]  VectorFormat=1-D array  Unit=A  AffineConversion=on
  idc/udc/cm : Scope  NumInputPorts=3
      settings: SampleTime=tc  ActiveDisplayYMinimum=-1357.19064  ActiveDisplayYMaximum=1822.38118
  ileg_dc_inv : nesl_utility/PS-Simulink Converter  PhysicalDomain=network_engine_domain  SubClassName=ps_output  LeftPortType=input  RightPortType=output  PseudoPeriodic=off  Frequencies=[]  VectorFormat=1-D array  Unit=A  AffineConversion=on
  sv_pwm : Subsystem
  switch_1 : Subsystem
      settings: PortSchema="{\"entries\":[{\"content\":{\"sides\":[{\"content\":{\"connectorIds\":[\"LConn1\"]},\"type\":\"ConnectorPlacement.EquallySpacedRectSide\",\"uuid\":\"9277da8d-d460-43e6-8478-dd662f15d226\"},{\"content\":{\"connectorIds\":[],\"side\":\"RIGHT\"},\"type\":\"ConnectorPlacement.EquallySpacedRectSide\",\"uuid\":\"a7ece396-f1d9-4f4f-a05b-db1fc65d6e1d\"},{\"content\":{\"connectorIds\":[\"LConn2\"],\"side\":\"TOP\"},\"type\":\"ConnectorPlacement.EquallySpacedRectSide\",\"uuid\":\"fdd70777-e9cf-4317-afb6-cae87f75d5b0\"},{\"content\":{\"connectorIds\":[\"RConn1\"],\"side\":\"BOTTOM\"},\"type\":\"ConnectorPlacement.EquallySpacedRectSide\",\"uuid\":\"2353ed68-b1a1-4775-9ca9-31e268d5443b\"}]},\"type\":\"ConnectorPlacement.EquallySpacedConnector\",\"uuid\":\"d5479f4c-4e65-4791-adcb-73df11f88590\"}],\"packageUris\":[\"http://schema.mathworks.com/mf0/Connector/R2020b\"],\"version\":\"1.0\"}"
  switch_2 : Subsystem
      settings: PortSchema="{\"entries\":[{\"content\":{\"sides\":[{\"content\":{\"connectorIds\":[\"LConn1\"]},\"type\":\"ConnectorPlacement.EquallySpacedRectSide\",\"uuid\":\"9277da8d-d460-43e6-8478-dd662f15d226\"},{\"content\":{\"connectorIds\":[],\"side\":\"RIGHT\"},\"type\":\"ConnectorPlacement.EquallySpacedRectSide\",\"uuid\":\"a7ece396-f1d9-4f4f-a05b-db1fc65d6e1d\"},{\"content\":{\"connectorIds\":[\"LConn2\"],\"side\":\"TOP\"},\"type\":\"ConnectorPlacement.EquallySpacedRectSide\",\"uuid\":\"fdd70777-e9cf-4317-afb6-cae87f75d5b0\"},{\"content\":{\"connectorIds\":[\"RConn1\"],\"side\":\"BOTTOM\"},\"type\":\"ConnectorPlacement.EquallySpacedRectSide\",\"uuid\":\"2353ed68-b1a1-4775-9ca9-31e268d5443b\"}]},\"type\":\"ConnectorPlacement.EquallySpacedConnector\",\"uuid\":\"d5479f4c-4e65-4791-adcb-73df11f88590\"}],\"packageUris\":[\"http://schema.mathworks.com/mf0/Connector/R2020b\"],\"version\":\"1.0\"}"
  switch_3 : Subsystem
      settings: PortSchema="{\"entries\":[{\"content\":{\"sides\":[{\"content\":{\"connectorIds\":[\"LConn1\"]},\"type\":\"ConnectorPlacement.EquallySpacedRectSide\",\"uuid\":\"9277da8d-d460-43e6-8478-dd662f15d226\"},{\"content\":{\"connectorIds\":[],\"side\":\"RIGHT\"},\"type\":\"ConnectorPlacement.EquallySpacedRectSide\",\"uuid\":\"a7ece396-f1d9-4f4f-a05b-db1fc65d6e1d\"},{\"content\":{\"connectorIds\":[\"LConn2\"],\"side\":\"TOP\"},\"type\":\"ConnectorPlacement.EquallySpacedRectSide\",\"uuid\":\"fdd70777-e9cf-4317-afb6-cae87f75d5b0\"},{\"content\":{\"connectorIds\":[\"RConn1\"],\"side\":\"BOTTOM\"},\"type\":\"ConnectorPlacement.EquallySpacedRectSide\",\"uuid\":\"2353ed68-b1a1-4775-9ca9-31e268d5443b\"}]},\"type\":\"ConnectorPlacement.EquallySpacedConnector\",\"uuid\":\"d5479f4c-4e65-4791-adcb-73df11f88590\"}],\"packageUris\":[\"http://schema.mathworks.com/mf0/Connector/R2020b\"],\"version\":\"1.0\"}"
  switch_4 : Subsystem
      settings: PortSchema="{\"entries\":[{\"content\":{\"sides\":[{\"content\":{\"connectorIds\":[\"LConn1\"]},\"type\":\"ConnectorPlacement.EquallySpacedRectSide\",\"uuid\":\"9277da8d-d460-43e6-8478-dd662f15d226\"},{\"content\":{\"connectorIds\":[],\"side\":\"RIGHT\"},\"type\":\"ConnectorPlacement.EquallySpacedRectSide\",\"uuid\":\"a7ece396-f1d9-4f4f-a05b-db1fc65d6e1d\"},{\"content\":{\"connectorIds\":[\"LConn2\"],\"side\":\"TOP\"},\"type\":\"ConnectorPlacement.EquallySpacedRectSide\",\"uuid\":\"fdd70777-e9cf-4317-afb6-cae87f75d5b0\"},{\"content\":{\"connectorIds\":[\"RConn1\"],\"side\":\"BOTTOM\"},\"type\":\"ConnectorPlacement.EquallySpacedRectSide\",\"uuid\":\"2353ed68-b1a1-4775-9ca9-31e268d5443b\"}]},\"type\":\"ConnectorPlacement.EquallySpacedConnector\",\"uuid\":\"d5479f4c-4e65-4791-adcb-73df11f88590\"}],\"packageUris\":[\"http://schema.mathworks.com/mf0/Connector/R2020b\"],\"version\":\"1.0\"}"
  switch_5 : Subsystem
      settings: PortSchema="{\"entries\":[{\"content\":{\"sides\":[{\"content\":{\"connectorIds\":[\"LConn1\"]},\"type\":\"ConnectorPlacement.EquallySpacedRectSide\",\"uuid\":\"9277da8d-d460-43e6-8478-dd662f15d226\"},{\"content\":{\"connectorIds\":[],\"side\":\"RIGHT\"},\"type\":\"ConnectorPlacement.EquallySpacedRectSide\",\"uuid\":\"a7ece396-f1d9-4f4f-a05b-db1fc65d6e1d\"},{\"content\":{\"connectorIds\":[\"LConn2\"],\"side\":\"TOP\"},\"type\":\"ConnectorPlacement.EquallySpacedRectSide\",\"uuid\":\"fdd70777-e9cf-4317-afb6-cae87f75d5b0\"},{\"content\":{\"connectorIds\":[\"RConn1\"],\"side\":\"BOTTOM\"},\"type\":\"ConnectorPlacement.EquallySpacedRectSide\",\"uuid\":\"2353ed68-b1a1-4775-9ca9-31e268d5443b\"}]},\"type\":\"ConnectorPlacement.EquallySpacedConnector\",\"uuid\":\"d5479f4c-4e65-4791-adcb-73df11f88590\"}],\"packageUris\":[\"http://schema.mathworks.com/mf0/Connector/R2020b\"],\"version\":\"1.0\"}"
  switch_6 : Subsystem
      settings: PortSchema="{\"entries\":[{\"content\":{\"sides\":[{\"content\":{\"connectorIds\":[\"LConn1\"]},\"type\":\"ConnectorPlacement.EquallySpacedRectSide\",\"uuid\":\"9277da8d-d460-43e6-8478-dd662f15d226\"},{\"content\":{\"connectorIds\":[],\"side\":\"RIGHT\"},\"type\":\"ConnectorPlacement.EquallySpacedRectSide\",\"uuid\":\"a7ece396-f1d9-4f4f-a05b-db1fc65d6e1d\"},{\"content\":{\"connectorIds\":[\"LConn2\"],\"side\":\"TOP\"},\"type\":\"ConnectorPlacement.EquallySpacedRectSide\",\"uuid\":\"fdd70777-e9cf-4317-afb6-cae87f75d5b0\"},{\"content\":{\"connectorIds\":[\"RConn1\"],\"side\":\"BOTTOM\"},\"type\":\"ConnectorPlacement.EquallySpacedRectSide\",\"uuid\":\"2353ed68-b1a1-4775-9ca9-31e268d5443b\"}]},\"type\":\"ConnectorPlacement.EquallySpacedConnector\",\"uuid\":\"d5479f4c-4e65-4791-adcb-73df11f88590\"}],\"packageUris\":[\"http://schema.mathworks.com/mf0/Connector/R2020b\"],\"version\":\"1.0\"}"
  udc : nesl_utility/PS-Simulink Converter  PhysicalDomain=network_engine_domain  SubClassName=ps_output  LeftPortType=input  RightPortType=output  PseudoPeriodic=off  Frequencies=[]  VectorFormat=1-D array  Unit=V  AffineConversion=on
  udc voltages : Scope  NumInputPorts=3
      settings: SampleTime=tc  ActiveDisplayYMinimum=71.02114  ActiveDisplayYMaximum=1379.58028
  us_a : PMIOPort  Side=Left
  us_b : PMIOPort  Port=2  Side=Left
  us_c : PMIOPort  Port=3  Side=Left
  Udc(+) : PMIOPort  Port=4  Side=Right
  Udc(-) : PMIOPort  Port=5  Side=Right
  tag scope: afe_mu_bottom=global, afe_mu_top=global, afe_mv_bottom=global, afe_mv_top=global, afe_mw_bottom=global, afe_mw_top=global, ic_dclink=global, ileg_dc_afe=global, udc=global
  wires:
  uab/1 -> sv_pwm/1(ab)
  [afe_mu_top] -> Simulink-PS Converter/1
  [afe_mu_bottom] -> Simulink-PS Converter1/1
  [afe_mv_top] -> Simulink-PS Converter2/1
  [afe_mv_bottom] -> Simulink-PS Converter3/1
  [afe_mw_top] -> Simulink-PS Converter4/1
  [afe_mw_bottom] -> Simulink-PS Converter5/1
  sv_pwm/1(firing_gates) -> Bus Selector/1
  Constant1/1 -> sv_pwm/2(enable)
  udc/1 -> [udc]  "udc"
  ic_dclink/1 -> [ic_dclink]
  ileg_dc_inv/1 -> [ileg_dc_afe]
  Step/1 -> Product5/1, Product4/1, Product3/1, Product2/1, Product/1, Product1/1
  Bus Selector/1 -> Product/2  "<pwm_afe_phase_u_top>"
  Bus Selector/2 -> Product1/2  "<pwm_afe_phase_u_bottom>"
  Bus Selector/3 -> Product2/2  "<pwm_afe_phase_v_top>"
  Bus Selector/4 -> Product3/2  "<pwm_afe_phase_v_bottom>"
  Bus Selector/5 -> Product4/2  "<pwm_afe_phase_w_top>"
  Bus Selector/6 -> Product5/2  "<pwm_afe_phase_w_bottom>"
  Product/1 -> [afe_mu_top]
  Product1/1 -> [afe_mu_bottom]
  Product2/1 -> [afe_mv_top]
  Product3/1 -> [afe_mv_bottom]
  Product4/1 -> [afe_mw_top]
  Product5/1 -> [afe_mw_bottom]
  [ic_dclink] -> idc/udc/cm/1  "ic_dclink"
  [udc] -> idc/udc/cm/2  "udc_dclink"
  Bus Creator/1 -> idc/udc/cm/3  "all_voltages_about_dclink"
  PS-Simulink Converter2/1 -> [udc_p_gnd], Bus Creator/1  "u_dclink_p_gnd"
  PS-Simulink Converter4/1 -> Bus Creator/2  "u_dclink_center_star_gnd"
  PS-Simulink Converter1/1 -> [udc_n_gnd], Bus Creator/3  "u_dclink_n_gnd"
  [udc_p_gnd] -> udc voltages/2  "udc(+) - gnd"
  [udc_n_gnd] -> udc voltages/3  "udc(-) - gnd"
  [udc] -> udc voltages/1  "udc(+) - udc(-)"
  connections:
  Current Sensor/LConn1 -- Udc(+)/RConn1 -- Voltage Sensor2/LConn1 -- Resistor/LConn1 -- Voltage Sensor3/LConn1 -- Current Sensor1/LConn1 -- switch_5/LConn2 -- switch_3/LConn2
  Udc(-)/RConn1 -- Capacitor/RConn1 -- Voltage Sensor2/RConn2 -- Resistor1/RConn1 -- Voltage Sensor1/LConn1 -- switch_2/RConn1 -- switch_6/RConn1 -- switch_4/RConn1
  switch_1/LConn1 -- Simulink-PS Converter/RConn1
  switch_2/LConn1 -- Simulink-PS Converter1/RConn1
  switch_3/LConn1 -- Simulink-PS Converter2/RConn1
  switch_4/LConn1 -- Simulink-PS Converter3/RConn1
  switch_5/LConn1 -- Simulink-PS Converter4/RConn1
  switch_6/LConn1 -- Simulink-PS Converter5/RConn1
  us_a/RConn1 -- switch_2/LConn2 -- switch_1/RConn1
  us_b/RConn1 -- switch_4/LConn2 -- switch_3/RConn1
  us_c/RConn1 -- switch_6/LConn2 -- switch_5/RConn1
  Voltage Sensor2/RConn1 -- udc/LConn1 -- dclink_measure/LConn1
  Current Sensor/RConn2 -- Capacitor/LConn1
  Current Sensor/RConn1 -- ic_dclink/LConn1
  switch_1/LConn2 -- Current Sensor1/RConn2
  Current Sensor1/RConn1 -- ileg_dc_inv/LConn1
  Resistor1/LConn1 -- Voltage Sensor/LConn1 -- Resistor/RConn1
  Voltage Sensor/RConn2 -- Electrical Reference/LConn1
  Voltage Sensor/RConn1 -- PS-Simulink Converter4/LConn1
  PS-Simulink Converter1/LConn1 -- Voltage Sensor1/RConn1
  Voltage Sensor1/RConn2 -- Electrical Reference1/LConn1
  PS-Simulink Converter2/LConn1 -- Voltage Sensor3/RConn1
  Voltage Sensor3/RConn2 -- Electrical Reference2/LConn1

== system afe_dq_inv_psm/afe_dq_inv_psm_mod1/afe_control ==
  Constant : Constant  Value=Vdc_norm_ref
  current_ctrl : Subsystem
  grid_current_sampling_and_alpha_beta_transformation : Subsystem
  grid_voltage_phase_lock_loops : Subsystem
  grid_voltage_sampling_and_alpha_beta_transformation : Subsystem
  i_alphabeta2xieta : Subsystem
  islanding_mode_detector : Subsystem
  udc_ctrl : Subsystem
  uab_out : Outport
  tag scope: ig_eta_pu=global, ig_xi_pu=global
  wires:
  Constant/1 -> udc_ctrl/2(udc_pu_ref)
  [vdc_pu] -> udc_ctrl/1(udc_pu)
  current_ctrl/1(uab_afe_out) -> uab_out/1
  udc_ctrl/1(i_xi_ref) -> current_ctrl/1(is_xi_ref)  "i_xi_ref"
  [gamma_grid_pll] -> islanding_mode_detector/1(gamma)
  [gamma_grid_pll] -> i_alphabeta2xieta/3(gamma)
  [vg_abc] -> grid_voltage_sampling_and_alpha_beta_transformation/1(v_abc)
  grid_voltage_sampling_and_alpha_beta_transformation/1(u_grid_alpha) -> islanding_mode_detector/2(alpha)
  grid_voltage_sampling_and_alpha_beta_transformation/2(u_grid_beta) -> islanding_mode_detector/3(beta)
  [ig_abc] -> grid_current_sampling_and_alpha_beta_transformation/1(i_abc)
  grid_current_sampling_and_alpha_beta_transformation/1(i_grid_alpha) -> i_alphabeta2xieta/1(alpha)
  grid_current_sampling_and_alpha_beta_transformation/2(i_grid_beta) -> i_alphabeta2xieta/2(beta)
  i_alphabeta2xieta/1(xi) -> [ig_xi_pu]
  i_alphabeta2xieta/2(v_grid_pos_eta) -> [ig_eta_pu]

== system afe_dq_inv_psm/afe_dq_inv_psm_mod1/brake ==
  Constant1 : Constant  Value=Vdc_ref
  Current Sensor3 : fl_lib/Electrical/Electrical Sensors/Current Sensor
  Integrator : Integrator
  MATLAB Function : MATLAB Function  TreatAsAtomicUnit=on  SystemSampleTime=ts_afe
  PS-Simulink Converter : nesl_utility/PS-Simulink Converter  PhysicalDomain=network_engine_domain  SubClassName=ps_output  LeftPortType=input  RightPortType=output  PseudoPeriodic=off  Frequencies=[]  VectorFormat=1-D array  Unit=V  AffineConversion=off
  Product : Product
  Product6 : Product
  Rbrake : Scope  NumInputPorts=2
      settings: SampleTime=tc  ActiveDisplayYMinimum=-1E-10  ActiveDisplayYMaximum=1.2E-9  DataLoggingVariableName=ScopeData2
  Resistor : fl_lib/Electrical/Electrical Elements/Resistor  R=4 Ohm  i_specify=off  i_priority=None  i=0 A  i_nominal_specify=off  i_nominal_value=1  i_nominal_unit=A  v_specify=off  v_priority=None  v=0 V  v_nominal_specify=off  v_nominal_value=1  v_nominal_unit=V
  Simulink-PS Converter4 : nesl_utility/Simulink-PS Converter  PhysicalDomain=network_engine_domain  SubClassName=ps_input  LeftPortType=input  RightPortType=output  PseudoPeriodic=off  Frequencies=[]  NoiseDistribution=none  NoiseParameters=[]  Unit=1  AffineConversion=on  FilteringAndDerivatives=provide  SimscapeFilterOrder=1  InputFilterTimeConstant=0.001  UdotUserProvided=0
  Step : Step  Time=time_aux_power_supply_fault  Before=1  After=0  SampleTime=0
  To Workspace1 : ToWorkspace  VariableName=energy_Rbrake_sim  SampleTime=ts_inv
      settings: MaxDataPoints=Ns_inv
  To Workspace10 : ToWorkspace  VariableName=power_Rbrake_sim  SampleTime=ts_inv
      settings: MaxDataPoints=Ns_inv
  Unit Delay : UnitDelay  SampleTime=ts_afe  HasFrameUpgradeWarning=on
  Voltage Sensor : fl_lib/Electrical/Electrical Sensors/Voltage Sensor
  Voltage Sensor1 : fl_lib/Electrical/Electrical Sensors/Voltage Sensor
  ibrakeR : nesl_utility/PS-Simulink Converter  PhysicalDomain=network_engine_domain  SubClassName=ps_output  LeftPortType=input  RightPortType=output  PseudoPeriodic=off  Frequencies=[]  VectorFormat=1-D array  Unit=A  AffineConversion=off
  switch_5 : Subsystem
      settings: PortSchema="{\"entries\":[{\"content\":{\"sides\":[{\"content\":{\"connectorIds\":[\"LConn1\"]},\"type\":\"ConnectorPlacement.EquallySpacedRectSide\",\"uuid\":\"9277da8d-d460-43e6-8478-dd662f15d226\"},{\"content\":{\"connectorIds\":[],\"side\":\"RIGHT\"},\"type\":\"ConnectorPlacement.EquallySpacedRectSide\",\"uuid\":\"a7ece396-f1d9-4f4f-a05b-db1fc65d6e1d\"},{\"content\":{\"connectorIds\":[\"LConn2\"],\"side\":\"TOP\"},\"type\":\"ConnectorPlacement.EquallySpacedRectSide\",\"uuid\":\"fdd70777-e9cf-4317-afb6-cae87f75d5b0\"},{\"content\":{\"connectorIds\":[\"RConn1\"],\"side\":\"BOTTOM\"},\"type\":\"ConnectorPlacement.EquallySpacedRectSide\",\"uuid\":\"2353ed68-b1a1-4775-9ca9-31e268d5443b\"}]},\"type\":\"ConnectorPlacement.EquallySpacedConnector\",\"uuid\":\"d5479f4c-4e65-4791-adcb-73df11f88590\"}],\"packageUris\":[\"http://schema.mathworks.com/mf0/Connector/R2020b\"],\"version\":\"1.0\"}"
  switch_6 : Subsystem
      settings: PortSchema="{\"entries\":[{\"content\":{\"sides\":[{\"content\":{},\"type\":\"ConnectorPlacement.EquallySpacedRectSide\",\"uuid\":\"9277da8d-d460-43e6-8478-dd662f15d226\"},{\"content\":{\"side\":\"RIGHT\"},\"type\":\"ConnectorPlacement.EquallySpacedRectSide\",\"uuid\":\"a7ece396-f1d9-4f4f-a05b-db1fc65d6e1d\"},{\"content\":{\"connectorIds\":[\"LConn1\"],\"side\":\"TOP\"},\"type\":\"ConnectorPlacement.EquallySpacedRectSide\",\"uuid\":\"fdd70777-e9cf-4317-afb6-cae87f75d5b0\"},{\"content\":{\"connectorIds\":[\"RConn1\"],\"side\":\"BOTTOM\"},\"type\":\"ConnectorPlacement.EquallySpacedRectSide\",\"uuid\":\"2353ed68-b1a1-4775-9ca9-31e268d5443b\"}]},\"type\":\"ConnectorPlacement.EquallySpacedConnector\",\"uuid\":\"d5479f4c-4e65-4791-adcb-73df11f88590\"}],\"packageUris\":[\"http://schema.mathworks.com/mf0/Connector/R2020b\"],\"version\":\"1.0\"}"
  ubrakeR : nesl_utility/PS-Simulink Converter  PhysicalDomain=network_engine_domain  SubClassName=ps_output  LeftPortType=input  RightPortType=output  PseudoPeriodic=off  Frequencies=[]  VectorFormat=1-D array  Unit=V  AffineConversion=off
  dc(+) : PMIOPort  Side=Left
  dc(-) : PMIOPort  Port=2  Side=Left
  tag scope: energy_Rbrake=global, power_Rbrake=global
  wires:
  Constant1/1 -> MATLAB Function/2(udc_ref)
  PS-Simulink Converter/1 -> MATLAB Function/1(u)
  MATLAB Function/1(y) -> Unit Delay/1
  ibrakeR/1 -> Product/1  "ibrakeR"
  ubrakeR/1 -> Product/2  "ubrakeR"
  Product/1 -> [power_Rbrake], Integrator/1
  Integrator/1 -> [energy_Rbrake]
  [power_Rbrake] -> Rbrake/1, To Workspace10/1  "power_Rbrake"
  [energy_Rbrake] -> Rbrake/2, To Workspace1/1  "energy_Rbrake"
  Step/1 -> Product6/1
  Unit Delay/1 -> Product6/2
  Product6/1 -> Simulink-PS Converter4/1
  connections:
  dc(-)/RConn1 -- switch_5/RConn1 -- Voltage Sensor/RConn2
  Voltage Sensor1/LConn1 -- Resistor/LConn1 -- Current Sensor3/RConn2
  PS-Simulink Converter/LConn1 -- Voltage Sensor/RConn1
  switch_5/LConn1 -- Simulink-PS Converter4/RConn1
  switch_6/RConn1 -- Voltage Sensor1/RConn2 -- Resistor/RConn1 -- switch_5/LConn2
  Voltage Sensor/LConn1 -- Current Sensor3/LConn1 -- switch_6/LConn1 -- dc(+)/RConn1
  Current Sensor3/RConn1 -- ibrakeR/LConn1
  Voltage Sensor1/RConn1 -- ubrakeR/LConn1
